simulink model "bpsk_rx8"  (Simulink 7.6)
settings: Solver=FixedStepDiscrete  StartTime=0.0  StopTime=1000  RelTol=1e-3
libraries: dsp_blocks x10, simulink x3
settings Model: Creator=Joshan  LastModifiedBy=Joshan

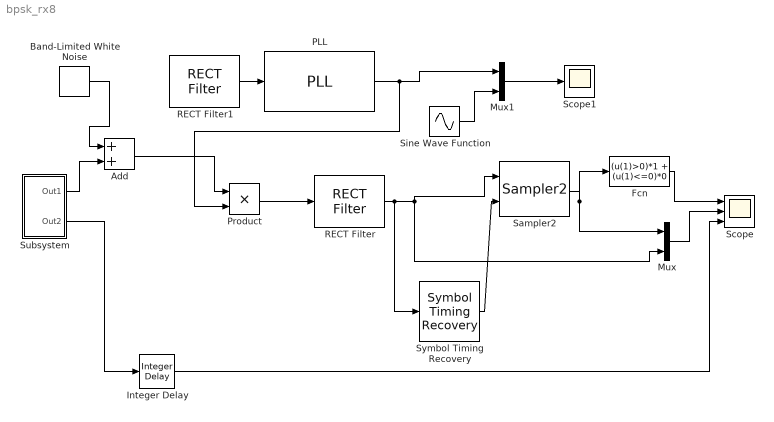
== system bpsk_rx8 ==
  Add : Sum
  Band-Limited White Noise : simulink/Sources/Band-Limited White Noise  SystemSampleTime=-1  Cov=[0.1]  Ts=1  seed=[23341]
  Fcn : Fcn  Expr=(u(1)>0)*1 + (u(1)<=0)*0
  Integer Delay : simulink/Discrete/Integer Delay  NumDelays=256  vinit=0.0  samptime=-1
  Mux : Mux  Inputs=2
  Mux1 : Mux  Inputs=2
  PLL : dsp_blocks/Timing /PLL  SystemSampleTime=-1  freq=0.05  freq_out=0.1  phi=0  amp=2  xi=1  K=2  T=200
  Product : Product  RndMeth=Zero
  RECT Filter : dsp_blocks/Filters/RECT Filter  SystemSampleTime=-1  f0=0  f1=0.1  filt_len=512
  RECT Filter1 : dsp_blocks/Filters/RECT Filter  SystemSampleTime=-1  f0=0.03  f1=0.07  filt_len=80
  Sampler2 : dsp_blocks/Conversions/Sampler2  SystemSampleTime=-1
  Scope : Scope  NumInputPorts=3
      settings: YMin=-5~-5~-5  YMax=5~5~5
  Scope1 : Scope
  Sine Wave Function : Sin  Amplitude=0.05  Frequency=2*pi*0.05  SampleTime=0
  Subsystem : Subsystem
  Symbol Timing Recovery : dsp_blocks/Timing /Symbol Timing Recovery  SystemSampleTime=-1  T=50  Tl=10000  tadj=1
  wires:
  Subsystem/2(Out2) -> Integer Delay/1
  Product/1 -> RECT Filter/1
  RECT Filter/1 -> Mux/2, Sampler2/1, Symbol Timing Recovery/1
  Fcn/1 -> Scope/1
  Mux/1 -> Scope/2
  Integer Delay/1 -> Scope/3
  Sampler2/1 -> Fcn/1, Mux/1
  RECT Filter1/1 -> PLL/1
  Mux1/1 -> Scope1/1
  PLL/1 -> Mux1/1, Product/2
  Sine Wave Function/1 -> Mux1/2
  Symbol Timing Recovery/1 -> Sampler2/2
  Add/1 -> Product/1
  Band-Limited White Noise/1 -> Add/1
  Subsystem/1(Out1) -> Add/2

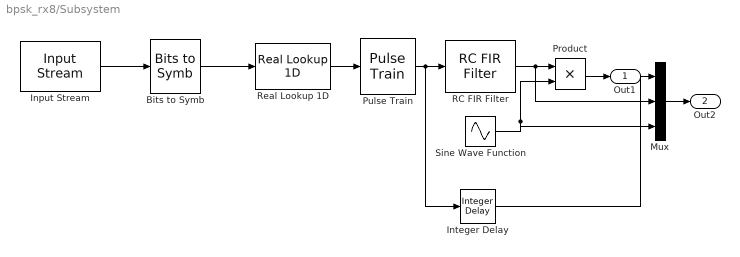
== system bpsk_rx8/Subsystem ==
  Bits to Symb : dsp_blocks/Conversions/Bits to Symb  SystemSampleTime=-1
  Input Stream : dsp_blocks/Sources//Sinks/Input Stream  SystemSampleTime=-1  period=10  width=1  fname=rand.mat
  Integer Delay : simulink/Discrete/Integer Delay  NumDelays=16  vinit=0.0  samptime=-1
  Mux : Mux  Inputs=3
  Product : Product  RndMeth=Zero
  Pulse Train : dsp_blocks/Conversions/Pulse Train  SystemSampleTime=-1  period=50
  RC FIR Filter : dsp_blocks/Filters/RC FIR Filter  SystemSampleTime=-1  period=10  beta=0.5  root=off  filt_len=128  win_type=on
  Real Lookup 1D : dsp_blocks/Conversions/Real Lookup 1D  SystemSampleTime=-1  table=[-1 1]
  Sine Wave Function : Sin  Frequency=2*pi*0.1  SampleTime=0
  Out1 : Outport
  Out2 : Outport  Port=2
  wires:
  Bits to Symb/1 -> Real Lookup 1D/1
  Input Stream/1 -> Bits to Symb/1
  Real Lookup 1D/1 -> Pulse Train/1
  Pulse Train/1 -> RC FIR Filter/1, Integer Delay/1
  RC FIR Filter/1 -> Product/1, Mux/2
  Sine Wave Function/1 -> Product/2, Mux/3
  Integer Delay/1 -> Mux/1
  Product/1 -> Out1/1
  Mux/1 -> Out2/1
